simulink model "Drone_2M_sim"  (R2022a)
settings: Solver=VariableStepAuto  StartTime=0.0  StopTime=SIM_TIME  RelTol=1e-3
undefined symbols (not defined in the file or in its folder): batteryMass, batVolt, body, deadCurrent, Dist, footZ, h1al, h1iuse, h1kp, h1td, h1ti, hoverControl, hoverVoltage, hval, hviuse, hvkp, hvtd, hvti, KDrag, Km, Ktrust, minimumMotorVolt, motorMass, paal, pakp, patd, pati, patiuse, pitch_act_lim, propellerMass, pval, pvkp, pvtd, pvti, pvtiuse, Ra, raal, rakp, ral, ratd, rati, ratiuse, rkp, roll_act_lim, roll_limit, rtd, rti, rtiuse, servoUs2Rad, sigbuilder_block, stepPitch, stepRoll, stepYaw, trust_lim, TubeMasse, TubeX, TubeY, UKp, ULimit, UTau_h ... (+49)
libraries: sm_lib x86, nesl_utility x39, sharedtransform x1
(part 1 of 4)
settings Model: Creator=Emar Manla  LastModifiedBy=User
settings DebuggingCC: UnconnectedInputMsg=warning  UnconnectedOutputMsg=warning  UnconnectedLineMsg=warning
settings RTWCC: DLArmComputeVersion=19.05

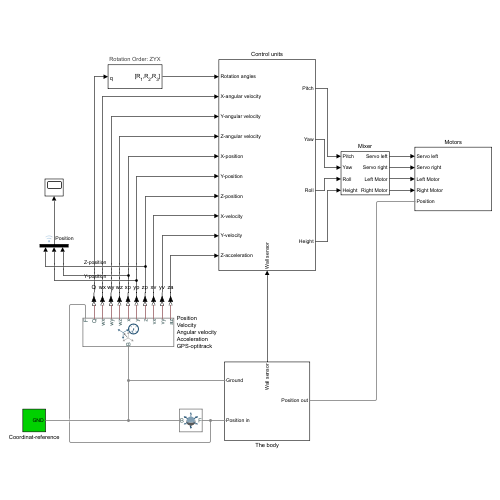
[thumbnail: Simulink's stored preview of the top-level diagram]
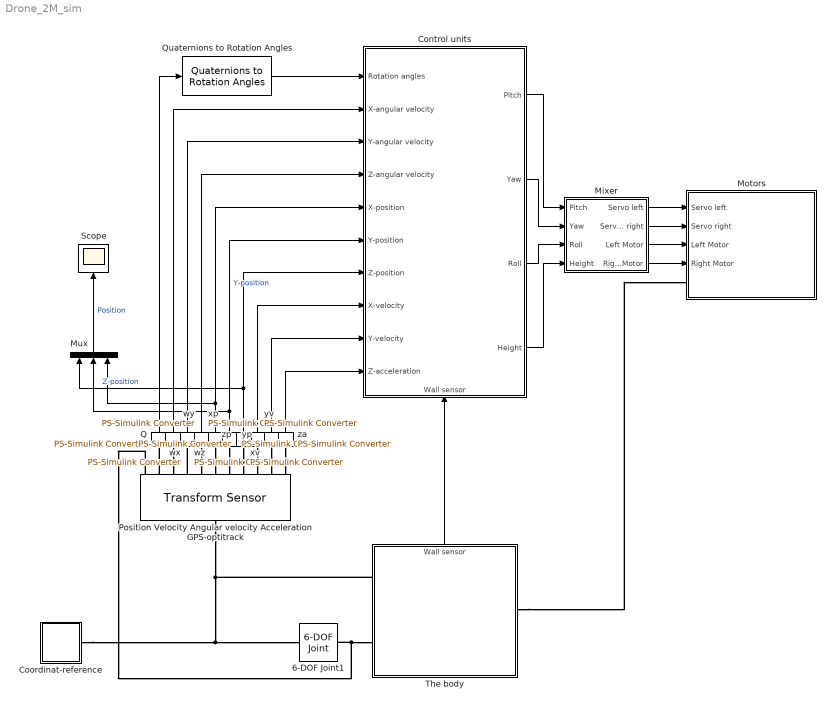
== system Drone_2M_sim ==
  6-DOF Joint1 : sm_lib/Joints/6-DOF Joint  JointMode=Normal  SenseConstraintForce=off  SenseConstraintForceX=off  SenseConstraintForceY=off  SenseConstraintForceZ=off  SenseConstraintTorque=off  SenseConstraintTorqueX=off  SenseConstraintTorqueY=off  SenseConstraintTorqueZ=off  SenseTotalForce=off  SenseTotalForceX=off  SenseTotalForceY=off  SenseTotalForceZ=off  SenseTotalTorque=off  SenseTotalTorqueX=off  SenseTotalTorqueY=off  SenseTotalTorqueZ=off  CompositeWrenchDir=FollowerOnBase  CompositeWrenchFrame=BaseFrame  PxEquilibriumPosition=0  PxEquilibriumPositionUnits=m  PxSpringStiffness=0  PxSpringStiffnessUnits=N/m  PxDampingCoefficient=0  PxDampingCoefficientUnits=N/(m/s)  PxTorqueActuationMode=NoTorque  PxMotionActuationMode=ComputedMotion  PxSensePosition=off  PxSenseVelocity=off  PxSenseAcceleration=off  PxSenseTorqueForce=off  PxSenseLowerLimitTorqueForce=off  PxSenseUpperLimitTorqueForce=off  PxLowerLimitSpecify=off  PxLowerLimitBound=-1  PxLowerLimitBoundUnits=m  PxLowerLimitStiffness=1e6  PxLowerLimitStiffnessUnits=N/m  PxLowerLimitDamping=1e3  PxLowerLimitDampingUnits=N/(m/s)  PxLowerLimitTransitionRegionWidth=1e-4  PxLowerLimitTransitionRegionWidthUnits=m  PxUpperLimitSpecify=off  PxUpperLimitBound=1  PxUpperLimitBoundUnits=m  PxUpperLimitStiffness=1e6  PxUpperLimitStiffnessUnits=N/m  PxUpperLimitDamping=1e3  PxUpperLimitDampingUnits=N/(m/s)  PxUpperLimitTransitionRegionWidth=1e-4  PxUpperLimitTransitionRegionWidthUnits=m  PxPositionTargetSpecify=off  PxPositionTargetPriority=High  PxPositionTargetValue=0  PxPositionTargetValueUnits=m  PxVelocityTargetSpecify=off  PxVelocityTargetPriority=High  PxVelocityTargetValue=0  PxVelocityTargetValueUnits=m/s  PyEquilibriumPosition=0  PyEquilibriumPositionUnits=m  PySpringStiffness=0  PySpringStiffnessUnits=N/m  PyDampingCoefficient=0  PyDampingCoefficientUnits=N/(m/s)  PyTorqueActuationMode=NoTorque  PyMotionActuationMode=ComputedMotion  PySensePosition=off  PySenseVelocity=off  PySenseAcceleration=off  PySenseTorqueForce=off  PySenseLowerLimitTorqueForce=off  PySenseUpperLimitTorqueForce=off  PyLowerLimitSpecify=off  PyLowerLimitBound=-1  PyLowerLimitBoundUnits=m  PyLowerLimitStiffness=1e6  PyLowerLimitStiffnessUnits=N/m  PyLowerLimitDamping=1e3  PyLowerLimitDampingUnits=N/(m/s)  PyLowerLimitTransitionRegionWidth=1e-4  PyLowerLimitTransitionRegionWidthUnits=m  PyUpperLimitSpecify=off  PyUpperLimitBound=1  PyUpperLimitBoundUnits=m  PyUpperLimitStiffness=1e6  PyUpperLimitStiffnessUnits=N/m  PyUpperLimitDamping=1e3  PyUpperLimitDampingUnits=N/(m/s)  PyUpperLimitTransitionRegionWidth=1e-4  PyUpperLimitTransitionRegionWidthUnits=m  PyPositionTargetSpecify=off  PyPositionTargetPriority=High  PyPositionTargetValue=0  PyPositionTargetValueUnits=m  PyVelocityTargetSpecify=off  PyVelocityTargetPriority=High  PyVelocityTargetValue=0  PyVelocityTargetValueUnits=m/s  PzEquilibriumPosition=0  PzEquilibriumPositionUnits=m  PzSpringStiffness=0  PzSpringStiffnessUnits=N/m  PzDampingCoefficient=0  PzDampingCoefficientUnits=N/(m/s)  PzTorqueActuationMode=NoTorque  PzMotionActuationMode=ComputedMotion  PzSensePosition=off  PzSenseVelocity=off  PzSenseAcceleration=off  PzSenseTorqueForce=off  PzSenseLowerLimitTorqueForce=off  PzSenseUpperLimitTorqueForce=off  PzLowerLimitSpecify=off  PzLowerLimitBound=-1  PzLowerLimitBoundUnits=m  PzLowerLimitStiffness=1e6  PzLowerLimitStiffnessUnits=N/m  PzLowerLimitDamping=1e3  PzLowerLimitDampingUnits=N/(m/s)  PzLowerLimitTransitionRegionWidth=1e-4  PzLowerLimitTransitionRegionWidthUnits=m  PzUpperLimitSpecify=off  PzUpperLimitBound=1  PzUpperLimitBoundUnits=m  PzUpperLimitStiffness=1e6  PzUpperLimitStiffnessUnits=N/m  PzUpperLimitDamping=1e3  PzUpperLimitDampingUnits=N/(m/s)  PzUpperLimitTransitionRegionWidth=1e-4  PzUpperLimitTransitionRegionWidthUnits=m  PzPositionTargetSpecify=off  PzPositionTargetPriority=High  PzPositionTargetValue=0  PzPositionTargetValueUnits=m  PzVelocityTargetSpecify=off  PzVelocityTargetPriority=High  PzVelocityTargetValue=0  PzVelocityTargetValueUnits=m/s  SphDefPosRotationMethod=None  SphDefPosRotationAngleUnits=deg  SphDefPosRotationStandardAxis=+Z  SphDefPosRotationAngle=0.0  SphDefPosRotationArbitraryAxis=[0 0 1]  SphDefPosFollAlignAxisA=+X  SphDefPosBaseAlignAxisA=+Y  SphDefPosFollAlignAxisB=+Y  SphDefPosBaseAlignAxisB=+Z  SphDefPosRotationSequenceAxes=FollowerAxes  SphDefPosRotationSequence=XYX  SphDefPosRotationSequenceAngles=[0 0 0]  SphDefPosRotationSequenceAnglesUnits=deg  SphDefPosRotationMatrix=[1 0 0; 0 1 0; 0 0 1]  SphEqPosRotationMethod=None  SphEqPosRotationAngleUnits=deg  SphEqPosRotationStandardAxis=+Z  SphEqPosRotationAngle=0.0  SphEqPosRotationArbitraryAxis=[0 0 1]  SphEqPosFollAlignAxisA=+X  SphEqPosBaseAlignAxisA=+Y  SphEqPosFollAlignAxisB=+Y  SphEqPosBaseAlignAxisB=+Z  SphEqPosRotationSequenceAxes=FollowerAxes  SphEqPosRotationSequence=XYX  SphEqPosRotationSequenceAngles=[0 0 0]  SphEqPosRotationSequenceAnglesUnits=deg  SphEqPosRotationMatrix=[1 0 0; 0 1 0; 0 0 1]  SphSpringStiffness=0  SphSpringStiffnessUnits=N*m/deg  SphDampingCoefficient=0  SphDampingCoefficientUnits=N*m/(deg/s)  SphActuateTorqueX=off  SphActuateTorqueY=off  SphActuateTorqueZ=off  SphActuateTorque=off  SphTorqueActuationMode=NoTorque  SphMotionActuationMode=ComputedMotion  SphActuationFrame=BaseFrame  SphSensePosition=off  SphSenseVelocityX=off  SphSenseVelocityY=off  SphSenseVelocityZ=off  SphSenseVelocity=off  SphSenseAccelerationX=off  SphSenseAccelerationY=off  SphSenseAccelerationZ=off  SphSenseAcceleration=off  SphSenseTorqueX=off  SphSenseTorqueY=off  SphSenseTorqueZ=off  SphSenseTorqueForce=off  SphSenseLowerLimitTorqueMag=off  SphSenseUpperLimitTorqueMag=off  SphSensingFrame=BaseFrame  SphLowerLimitSpecify=off  SphLowerLimitBound=15  SphLowerLimitBoundUnits=deg  SphLowerLimitStiffness=1e4  SphLowerLimitStiffnessUnits=N*m/deg  SphLowerLimitDamping=10  SphLowerLimitDampingUnits=N*m/(deg/s)  SphLowerLimitTransitionRegionWidth=0.1  SphLowerLimitTransitionRegionWidthUnits=deg  SphUpperLimitSpecify=off  SphUpperLimitBound=45  SphUpperLimitBoundUnits=deg  SphUpperLimitStiffness=1e4  SphUpperLimitStiffnessUnits=N*m/deg  SphUpperLimitDamping=10  SphUpperLimitDampingUnits=N*m/(deg/s)  SphUpperLimitTransitionRegionWidth=0.1  SphUpperLimitTransitionRegionWidthUnits=deg  SphPositionTargetRotationMethod=None  SphPositionTargetRotationAngleUnits=deg  SphPositionTargetRotationStandardAxis=+Z  SphPositionTargetRotationAngle=0.0  SphPositionTargetRotationArbitraryAxis=[0 0 1]  SphPositionTargetFollAlignAxisA=+X  SphPositionTargetBaseAlignAxisA=+Y  SphPositionTargetFollAlignAxisB=+Y  SphPositionTargetBaseAlignAxisB=+Z  SphPositionTargetRotationSequenceAxes=FollowerAxes  SphPositionTargetRotationSequence=XYX  SphPositionTargetRotationSequenceAngles=[0 0 0]  SphPositionTargetRotationSequenceAnglesUnits=deg  SphPositionTargetRotationMatrix=[1 0 0; 0 1 0; 0 0 1]  SphPositionTargetSpecify=off  SphPositionTargetPriority=High  SphVelocityTargetValue=[0 0 0]  SphVelocityTargetValueUnits=deg/s  SphVelocityTargetSpecify=off  SphVelocityTargetPriority=High  SphVelocityTargetInFollowerFrame=on
  Control units : Subsystem
      settings: PortSchema="{\"entries\":[{\"content\":{\"sides\":[{\"content\":{\"connectorIds\":[\"In1\",\"In2\",\"In3\",\"In4\",\"In5\",\"In6\",\"In7\",\"In8\",\"In9\",\"In10\"]},\"type\":\"ConnectorPlacement.EquallySpacedRectSide\",\"uuid\":\"d340103e-df0a-4210-bd7d-281fdd84635a\"},{\"content\":{\"connectorIds\":[\"Out1\",\"Out2\",\"Out3\",\"Out4\"],\"side\":\"RIGHT\"},\"type\":\"ConnectorPlacement.EquallySpacedRectSide\",\"uuid\":\"102c7985-49c9-4d2d-a8bd-e75b65b3747e\"},{\"content\":{\"connectorIds\":[],\"side\":\"TOP\"},\"type\":\"ConnectorPlacement.EquallySpacedRectSide\",\"uuid\":\"91d195dd-fb46-4973-a33d-9a570104b146\"},{\"content\":{\"connectorIds\":[\"In11\"],\"side\":\"BOTTOM\"},\"type\":\"ConnectorPlacement.EquallySpacedRectSide\",\"uuid\":\"6514ae44-da82-47f0-9c16-8828a99121c7\"}]},\"type\":\"ConnectorPlacement.EquallySpacedConnector\",\"uuid\":\"d6f0110d-ada7-4d6d-ac5d-6be58cf7ad12\"}],\"packageUris\":[\"http://schema.mathworks.com/mf0/Connector/R2020b\"],\"version\":\"1.0\"}"
  Coordinat-reference : Subsystem
  Mixer : Subsystem
  Motors : Subsystem
  Mux : Mux  Inputs=3
  Position Velocity Angular velocity Acceleration GPS-optitrack : sm_lib/Frames and Transforms/Transform Sensor  MeasurementFrame=World  SenseAngle=off  SenseAxis=off  SenseAngle1=off  SenseAngle2=off  SenseAngle3=off  SenseQ=on  SenseR=off  SenseOmegaX=on  SenseOmegaY=on  SenseOmegaZ=on  SenseOmega1=off  SenseOmega2=off  SenseOmega3=off  SenseQDot=off  SenseRDot=off  SenseAlphaX=off  SenseAlphaY=off  SenseAlphaZ=off  SenseAlpha1=off  SenseAlpha2=off  SenseAlpha3=off  SenseQDDot=off  SenseRDDot=off  SenseX=on  SenseY=on  SenseZ=on  SenseRad=off  SenseAzim=off  SenseDist=off  SenseInc=off  SenseXDot=on  SenseYDot=on  SenseZDot=off  SenseRadDot=off  SenseAzimDot=off  SenseDistDot=off  SenseIncDot=off  SenseXDDot=off  SenseYDDot=off  SenseZDDot=on  SenseRadDDot=off  SenseAzimDDot=off  SenseDistDDot=off  SenseIncDDot=off
  Q : nesl_utility/PS-Simulink Converter  PhysicalDomain=network_engine_domain  SubClassName=ps_output  LeftPortType=input  RightPortType=output  PseudoPeriodic=off  Frequencies=[]  VectorFormat=1-D array  Unit=inherit  AffineConversion=off
      settings: SourceProductBaseCode=SS,PW,VE
  Quaternions to Rotation Angles : sharedtransform/Quaternions to Rotation Angles  rotationOrder=ZYX  aMode=aMode
      settings: SourceProductBaseCode=AE,PW,DR,MT,VE
  Scope : Scope
  The body : Subsystem
      settings: PortSchema="{\"entries\":[{\"content\":{\"sides\":[{\"content\":{\"connectorIds\":[\"LConn1\",\"LConn2\"]},\"type\":\"ConnectorPlacement.EquallySpacedRectSide\",\"uuid\":\"ab37280a-1c0d-4698-b613-0144e6e2cacd\"},{\"content\":{\"connectorIds\":[\"RConn1\"],\"side\":\"RIGHT\"},\"type\":\"ConnectorPlacement.EquallySpacedRectSide\",\"uuid\":\"d03955d5-50d7-455a-845d-681fe8b68e0b\"},{\"content\":{\"connectorIds\":[\"Out1\"],\"side\":\"TOP\"},\"type\":\"ConnectorPlacement.EquallySpacedRectSide\",\"uuid\":\"5fdb51a7-fdf2-45ed-bb3d-bc4d58960f05\"}]},\"type\":\"ConnectorPlacement.EquallySpacedConnector\",\"uuid\":\"890992e6-4a83-43bc-854b-607ea4381fcf\"}],\"packageUris\":[\"http://schema.mathworks.com/mf0/Connector/R2020b\"],\"version\":\"1.0\"}"
  wx : nesl_utility/PS-Simulink Converter  PhysicalDomain=network_engine_domain  SubClassName=ps_output  LeftPortType=input  RightPortType=output  PseudoPeriodic=off  Frequencies=[]  VectorFormat=1-D array  Unit=inherit  AffineConversion=off
      settings: SourceProductBaseCode=SS,PW,VE
  wy : nesl_utility/PS-Simulink Converter  PhysicalDomain=network_engine_domain  SubClassName=ps_output  LeftPortType=input  RightPortType=output  PseudoPeriodic=off  Frequencies=[]  VectorFormat=1-D array  Unit=inherit  AffineConversion=off
      settings: SourceProductBaseCode=SS,PW,VE
  wz : nesl_utility/PS-Simulink Converter  PhysicalDomain=network_engine_domain  SubClassName=ps_output  LeftPortType=input  RightPortType=output  PseudoPeriodic=off  Frequencies=[]  VectorFormat=1-D array  Unit=inherit  AffineConversion=off
      settings: SourceProductBaseCode=SS,PW,VE
  xp : nesl_utility/PS-Simulink Converter  PhysicalDomain=network_engine_domain  SubClassName=ps_output  LeftPortType=input  RightPortType=output  PseudoPeriodic=off  Frequencies=[]  VectorFormat=1-D array  Unit=inherit  AffineConversion=off
      settings: SourceProductBaseCode=SS,PW,VE
  xv : nesl_utility/PS-Simulink Converter  PhysicalDomain=network_engine_domain  SubClassName=ps_output  LeftPortType=input  RightPortType=output  PseudoPeriodic=off  Frequencies=[]  VectorFormat=1-D array  Unit=inherit  AffineConversion=off
      settings: SourceProductBaseCode=SS,PW,VE
  yp : nesl_utility/PS-Simulink Converter  PhysicalDomain=network_engine_domain  SubClassName=ps_output  LeftPortType=input  RightPortType=output  PseudoPeriodic=off  Frequencies=[]  VectorFormat=1-D array  Unit=inherit  AffineConversion=off
      settings: SourceProductBaseCode=SS,PW,VE
  yv : nesl_utility/PS-Simulink Converter  PhysicalDomain=network_engine_domain  SubClassName=ps_output  LeftPortType=input  RightPortType=output  PseudoPeriodic=off  Frequencies=[]  VectorFormat=1-D array  Unit=inherit  AffineConversion=off
      settings: SourceProductBaseCode=SS,PW,VE
  za : nesl_utility/PS-Simulink Converter  PhysicalDomain=network_engine_domain  SubClassName=ps_output  LeftPortType=input  RightPortType=output  PseudoPeriodic=off  Frequencies=[]  VectorFormat=1-D array  Unit=inherit  AffineConversion=off
      settings: SourceProductBaseCode=SS,PW,VE
  zp : nesl_utility/PS-Simulink Converter  PhysicalDomain=network_engine_domain  SubClassName=ps_output  LeftPortType=input  RightPortType=output  PseudoPeriodic=off  Frequencies=[]  VectorFormat=1-D array  Unit=inherit  AffineConversion=off
      settings: SourceProductBaseCode=SS,PW,VE
  wires:
  Q/1 -> Quaternions to Rotation Angles/1
  Mixer/1(Servo left) -> Motors/1(Servo left)
  Mixer/2(Servo right) -> Motors/2(Servo right)
  Mixer/3(Left Motor) -> Motors/3(Left Motor)
  Mixer/4(Right Motor) -> Motors/4(Right Motor)
  Quaternions to Rotation Angles/1 -> Control units/1(Rotation angles)
  xp/1 -> Mux/3, Control units/5(X-position)
  yp/1 -> Mux/2, Control units/6(Y-position)  "Y-position"
  zp/1 -> Mux/1, Control units/7(Z-position)  "Z-position"
  xv/1 -> Control units/8(X-velocity)
  yv/1 -> Control units/9(Y-velocity)
  za/1 -> Control units/10(Z-acceleration)
  wx/1 -> Control units/2(X-angular velocity)
  wy/1 -> Control units/3(Y-angular velocity)
  wz/1 -> Control units/4(Z-angular velocity)
  The body/1(Wall sensor) -> Control units/11(Wall sensor)
  Control units/1(Pitch) -> Mixer/1(Pitch)
  Control units/2(Yaw) -> Mixer/2(Yaw)
  Control units/3(Roll) -> Mixer/3(Roll)
  Control units/4(Height) -> Mixer/4(Height)
  Mux/1 -> Scope/1  "Position"
  connections:
  wx/LConn1 -- Position Velocity Angular velocity Acceleration GPS-optitrack/RConn3
  Position Velocity Angular velocity Acceleration GPS-optitrack/RConn2 -- Q/LConn1
  wz/LConn1 -- Position Velocity Angular velocity Acceleration GPS-optitrack/RConn5
  Position Velocity Angular velocity Acceleration GPS-optitrack/RConn4 -- wy/LConn1
  xp/LConn1 -- Position Velocity Angular velocity Acceleration GPS-optitrack/RConn6
  yp/LConn1 -- Position Velocity Angular velocity Acceleration GPS-optitrack/RConn7
  xv/LConn1 -- Position Velocity Angular velocity Acceleration GPS-optitrack/RConn9
  yv/LConn1 -- Position Velocity Angular velocity Acceleration GPS-optitrack/RConn10
  Position Velocity Angular velocity Acceleration GPS-optitrack/LConn1 -- The body/LConn1 -- Coordinat-reference/RConn1 -- 6-DOF Joint1/LConn1
  Position Velocity Angular velocity Acceleration GPS-optitrack/RConn1 -- The body/LConn2 -- 6-DOF Joint1/RConn1
  The body/RConn1 -- Motors/LConn1
  zp/LConn1 -- Position Velocity Angular velocity Acceleration GPS-optitrack/RConn8
  za/LConn1 -- Position Velocity Angular velocity Acceleration GPS-optitrack/RConn11

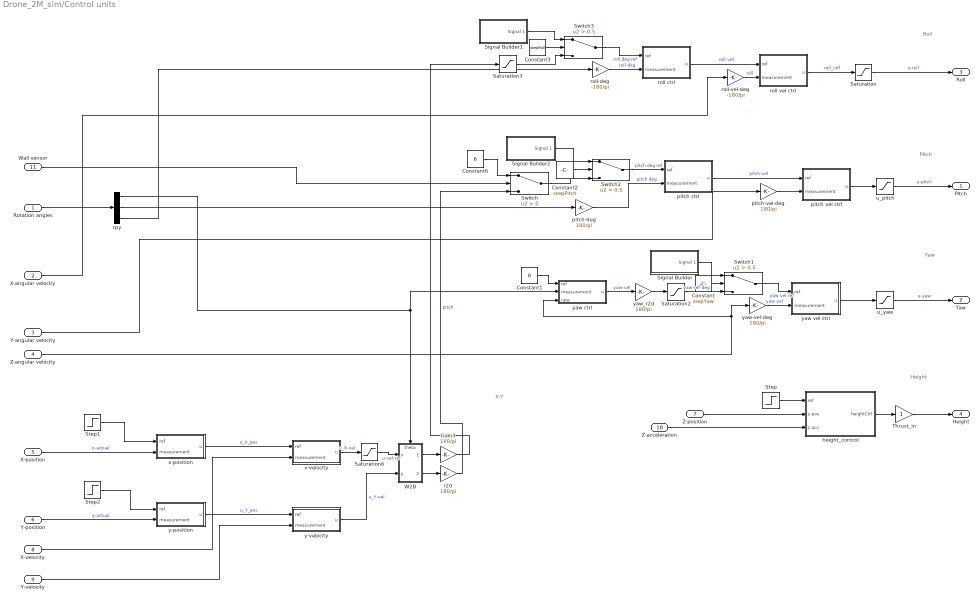
== system Drone_2M_sim/Control units ==
  note: Pitch
  note: Yaw
  note: Roll
  note: Height
  note: X-Y
  Rotation angles : Inport
  X-angular velocity : Inport  Port=2
  Y-angular velocity : Inport  Port=3
  Z-angular velocity : Inport  Port=4
  X-position : Inport  Port=5
  Y-position : Inport  Port=6
  Z-position : Inport  Port=7
  X-velocity : Inport  Port=8
  Y-velocity : Inport  Port=9
  Z-acceleration : Inport  Port=10
  Wall sensor : Inport  Port=11
  Constant : Constant  Value=stepYaw
  Constant1 : Constant  Value=0
  Constant2 : Constant  Value=stepPitch
  Constant3 : Constant  Value=stepRoll
  Constant6 : Constant  Value=6
  Gain3 : Gain  Gain=180/pi
  Saturation : Saturate  UpperLimit=roll_act_lim  LowerLimit=-roll_act_lim
  Saturation2 : Saturate  UpperLimit=yaw_rate_limit  LowerLimit=-yaw_rate_limit
  Saturation3 : Saturate  UpperLimit=roll_limit  LowerLimit=-roll_limit
  Saturation6 : Saturate  UpperLimit=0.008  LowerLimit=-0.008
  Signal Builder : Subsystem  Tag=STV Subsys  LoadFcn=sigbuilder_block('load');  StartFcn=sigbuilder_block('start');  StopFcn=sigbuilder_block('stop');  ClipboardFcn=sigbuilder_block('clipboard');  mask(Sigbuilder block){tuvar=[0:10]}
      mask help: Simulink:masks:SigbuilderBlock_MD
      mask init:
      | if ~strcmp(get_param(bdroot(gcbh),'SimulationStatus'),'stopped') tuvar = sigbuilder_block('maskInit'); end
      settings: CopyFcn=sigbuilder_block('copy');  DeleteFcn=sigbuilder_block('delete');  ModelCloseFcn=sigbuilder_block('modelClose');  PreSaveFcn=sigbuilder_block('preSave');  PauseFcn=sigbuilder_block('pause');  ContinueFcn=sigbuilder_block('continue');  NameChangeFcn=sigbuilder_block('namechange');  OpenFcn=sigbuilder_block('open',[310.5 301 644 239 ]);  CloseFcn=sigbuilder_block('close');
      mask Display: plot(0, 0, 100, 100,[2, 2, 32, 32, 2], [68, 8, 8, 68, 68],[32, 2], [38, 38], [32, 19, 2],[53, 60, 44], [32, 17, 17, 2],[16, 16, 31, 31]);txt = getActiveGroup(gcbh);text(2, 100, txt,'verticalAlignment', 'top');
  Signal Builder1 : Subsystem  Tag=STV Subsys  LoadFcn=sigbuilder_block('load');  StartFcn=sigbuilder_block('start');  StopFcn=sigbuilder_block('stop');  ClipboardFcn=sigbuilder_block('clipboard');  mask(Sigbuilder block){tuvar=[0:10]}
      mask help: Simulink:masks:SigbuilderBlock_MD
      mask init:
      | if ~strcmp(get_param(bdroot(gcbh),'SimulationStatus'),'stopped') tuvar = sigbuilder_block('maskInit'); end
      settings: CopyFcn=sigbuilder_block('copy');  DeleteFcn=sigbuilder_block('delete');  ModelCloseFcn=sigbuilder_block('modelClose');  PreSaveFcn=sigbuilder_block('preSave');  PauseFcn=sigbuilder_block('pause');  ContinueFcn=sigbuilder_block('continue');  NameChangeFcn=sigbuilder_block('namechange');  OpenFcn=sigbuilder_block('open',[310.5 301 644 239 ]);  CloseFcn=sigbuilder_block('close');
      mask Display: plot(0, 0, 100, 100,[2, 2, 32, 32, 2], [68, 8, 8, 68, 68],[32, 2], [38, 38], [32, 19, 2],[53, 60, 44], [32, 17, 17, 2],[16, 16, 31, 31]);txt = getActiveGroup(gcbh);text(2, 100, txt,'verticalAlignment', 'top');
  Signal Builder2 : Subsystem  Tag=STV Subsys  LoadFcn=sigbuilder_block('load');  StartFcn=sigbuilder_block('start');  StopFcn=sigbuilder_block('stop');  ClipboardFcn=sigbuilder_block('clipboard');  mask(Sigbuilder block){tuvar=[0:10]}
      mask help: Simulink:masks:SigbuilderBlock_MD
      mask init:
      | if ~strcmp(get_param(bdroot(gcbh),'SimulationStatus'),'stopped') tuvar = sigbuilder_block('maskInit'); end
      settings: CopyFcn=sigbuilder_block('copy');  DeleteFcn=sigbuilder_block('delete');  ModelCloseFcn=sigbuilder_block('modelClose');  PreSaveFcn=sigbuilder_block('preSave');  PauseFcn=sigbuilder_block('pause');  ContinueFcn=sigbuilder_block('continue');  NameChangeFcn=sigbuilder_block('namechange');  OpenFcn=sigbuilder_block('open',[310.5 301 644 239 ]);  CloseFcn=sigbuilder_block('close');
      mask Display: plot(0, 0, 100, 100,[2, 2, 32, 32, 2], [68, 8, 8, 68, 68],[32, 2], [38, 38], [32, 19, 2],[53, 60, 44], [32, 17, 17, 2],[16, 16, 31, 31]);txt = getActiveGroup(gcbh);text(2, 100, txt,'verticalAlignment', 'top');
  Step : Step  Time=z_steptime  After=z_ref  SampleTime=0
  Step1 : Step  Time=x_steptime  After=x_ref  SampleTime=0
  Step2 : Step  Time=y_steptime  After=y_ref  SampleTime=0
  Switch : Switch  Criteria=u2 > Threshold  SaturateOnIntegerOverflow=off  InputSameDT=off
  Switch1 : Switch  Criteria=u2 > Threshold  Threshold=0.5  SaturateOnIntegerOverflow=off  InputSameDT=off
  Switch2 : Switch  Criteria=u2 > Threshold  Threshold=0.5  SaturateOnIntegerOverflow=off  InputSameDT=off
  Switch3 : Switch  Criteria=u2 > Threshold  Threshold=0.5  SaturateOnIntegerOverflow=off  InputSameDT=off
  Thrust_in : Gain
  W2B : Subsystem
      settings: PortSchema="{\"entries\":[{\"content\":{\"sides\":[{\"content\":{\"connectorIds\":[\"In1\",\"In2\"]},\"type\":\"ConnectorPlacement.EquallySpacedRectSide\",\"uuid\":\"cbb8a801-9e3d-4042-a15f-2b3de221b3e9\"},{\"content\":{\"connectorIds\":[\"Out1\",\"Out2\"],\"side\":\"RIGHT\"},\"type\":\"ConnectorPlacement.EquallySpacedRectSide\",\"uuid\":\"345cd2b8-58a5-4721-b50a-def58b68f03f\"},{\"content\":{\"connectorIds\":[\"In3\"],\"side\":\"TOP\"},\"type\":\"ConnectorPlacement.EquallySpacedRectSide\",\"uuid\":\"a136db43-a3b7-4cbd-bccf-57f3512c0ab6\"}]},\"type\":\"ConnectorPlacement.EquallySpacedConnector\",\"uuid\":\"f3e3d7e3-47e2-471e-9ab4-460d41ed2370\"}],\"packageUris\":[\"http://schema.mathworks.com/mf0/Connector/R2020b\"],\"version\":\"1.0\"}"
  height_control : Subsystem
  pitch ctrl : Subsystem
  pitch vel ctrl : Subsystem
  pitch-deg : Gain  Gain=180/pi
  pitch-vel-deg : Gain  Gain=180/pi
  r2d : Gain  Gain=180/pi
  roll ctrl : Subsystem
  roll vel ctrl : Subsystem
  roll-deg : Gain  Gain=-180/pi
  roll-vel-deg : Gain  Gain=-180/pi
  rpy : Demux  Outputs=3
  u_pitch : Saturate  UpperLimit=pitch_act_lim  LowerLimit=-pitch_act_lim
  u_yaw : Saturate  UpperLimit=yaw_act_lim  LowerLimit=-yaw_act_lim
  x-position : Subsystem
  x-velocity : Subsystem
  y-position : Subsystem
  y-velocity : Subsystem
  yaw ctrl : Subsystem
  yaw vel ctrl : Subsystem
  yaw-vel-deg : Gain  Gain=180/pi
  yaw_r2d : Gain  Gain=180/pi
  Pitch : Outport
  Yaw : Outport  Port=2
  Roll : Outport  Port=3
  Height : Outport  Port=4
  wires:
  Wall sensor/1 -> Switch/2
  pitch-vel-deg/1 -> pitch vel ctrl/2(measurement)
  Step/1 -> height_control/1(ref)
  pitch ctrl/1(u) -> pitch vel ctrl/1(ref)  "pitch-vel"
  rpy/3 -> roll-deg/1
  x-velocity/1(u) -> Saturation6/1  "u_X-vel"
  roll-deg/1 -> roll ctrl/2(measurement)  "roll deg"
  y-position/1(u) -> y-velocity/1(ref)  "u_Y_pos"
  yaw vel ctrl/1(u) -> u_yaw/1
  Saturation6/1 -> W2B/1(x)  "u-vel-ref"
  u_yaw/1 -> Yaw/1  "u-yaw"
  Gain3/1 -> Saturation3/1
  r2d/1 -> Switch/3  "pitch"
  Y-position/1 -> y-position/2(measurement)  "y-actual"
  roll ctrl/1(u) -> roll vel ctrl/1(ref)  "roll-vel"
  u_pitch/1 -> Pitch/1  "u-pitch"
  Saturation/1 -> Roll/1  "u-roll"
  roll-vel-deg/1 -> roll vel ctrl/2(measurement)  "roll"
  x-position/1(u) -> x-velocity/1(ref)  "u_X_pos"
  pitch-deg/1 -> pitch ctrl/2(measurement)  "pitch deg"
  height_control/1(heightCtrl) -> Thrust_in/1
  Constant6/1 -> Switch/1
  roll vel ctrl/1(u) -> Saturation/1  "roll_ctrl"
  Y-velocity/1 -> y-velocity/2(measurement)
  Step2/1 -> y-position/1(ref)
  yaw-vel-deg/1 -> yaw vel ctrl/2(measurement)  "yaw vel"
  rpy/1 -> W2B/3(theta), yaw ctrl/2(measurement)
  yaw ctrl/1(u) -> yaw_r2d/1  "yaw-vel"
  Z-position/1 -> height_control/2(z-pos)
  rpy/2 -> pitch-deg/1
  Y-angular velocity/1 -> pitch-vel-deg/1
  Z-angular velocity/1 -> yaw ctrl/3(rate), yaw-vel-deg/1
  W2B/1(roll) -> Gain3/1
  X-angular velocity/1 -> roll-vel-deg/1
  y-velocity/1(u) -> W2B/2(y)  "u_Y-vel"
  W2B/2(pitch) -> r2d/1
  X-velocity/1 -> x-velocity/2(measurement)
  Z-acceleration/1 -> height_control/3(z-acc)
  pitch vel ctrl/1(u) -> u_pitch/1
  X-position/1 -> x-position/2(measurement)  "x-actual"
  Step1/1 -> x-position/1(ref)
  yaw_r2d/1 -> Saturation2/1
  Rotation angles/1 -> rpy/1
  Thrust_in/1 -> Height/1
  Constant1/1 -> yaw ctrl/1(ref)
  Switch1/1 -> yaw vel ctrl/1(ref)  "yaw vel ref"
  Saturation2/1 -> Switch1/3  "yaw-ref-deg"
  Signal Builder/1(Signal 1) -> Switch1/1
  Saturation3/1 -> Switch3/3
  Signal Builder1/1(Signal 1) -> Switch3/1
  Switch/1 -> Switch2/3
  Switch2/1 -> pitch ctrl/1(ref)  "pitch deg ref"
  Signal Builder2/1(Signal 1) -> Switch2/1
  Constant/1 -> Switch1/2
  Constant2/1 -> Switch2/2
  Constant3/1 -> Switch3/2
  Switch3/1 -> roll ctrl/1(ref)  "roll deg ref"

== system Drone_2M_sim/Coordinat-reference ==
  GroundT : sm_lib/Frames and Transforms/Rigid Transform  TranslationMethod=Cartesian  TranslationStandardOffset=0  TranslationLengthUnit=m  TranslationStandardAxis=+Z  TranslationCartesianOffset=[0 0 0]  TranslationROffset=0  TranslationROffsetUnits=m  TranslationZOffset=0  TranslationZOffsetUnits=m  TranslationThetaOffset=0  TranslationThetaOffsetUnits=deg  RotationMethod=None  RotationAngleUnits=deg  RotationStandardAxis=+Z  RotationAngle=0.0  RotationArbitraryAxis=[0 0 1]  FollAlignAxisA=+X  BaseAlignAxisA=+Y  FollAlignAxisB=+Y  BaseAlignAxisB=+Z  RotationSequenceAxes=FollowerAxes  RotationSequence=XYX  RotationSequenceAngles=[0 0 0]  RotationSequenceAnglesUnits=deg  RotationMatrix=[1 0 0; 0 1 0; 0 0 1]
  Mechanism Configuration : sm_lib/Utilities/Mechanism Configuration  UniformGravity=Constant  GravityVector=[0 0 -9.82]  GravityUnits=m/s^2  LinearizationDelta=0.001  JointModeTransitionNonlinearIterations=2
  Solver Configuration : nesl_utility/Solver Configuration  PhysicalDomain=network_engine_domain  SubClassName=solver  LeftPortType=input  RightPortType=generic  Tones=[]  Harmonics=[]  SimulateNoise=off  Profile=off  UseLocalSampling=off  EnableSwitchedLinearOptims=on  FrequencyDomain=off  UseCCode=off  RelTol=0.001  AbsTol=1e-06  MinStep=1e-09  ToWorkspace=off  RevertToSquareIcSolve=off  NumHomotopyIterations=100  PhasorMode=off  PhasorModeNumHarmonics=1  IndexReductionMethod=DerivativeReplacement  DoDC=off  ResidualTolerance=1e-09  UseLocalSolver=off  LocalSolverChoice=NE_BACKWARD_EULER_ADVANCER  LocalSolverSampleTime=0.001  DoFixedCost=off  MaxNonlinIter=3  MaxModeIter=2  ComputeImpulses=off  ImpulseIterations=2  LinearAlgebra=Sparse  LinearAlgebraNumThread=0  EquationFormulation=NE_TIME_EF  DelaysMemoryBudget=1024  AutomaticFiltering=on  FilteringTimeConstant=0.001  PartitionStorageMethod=AS_NEEDED  PartitionMemoryBudget=1024  PartitionMethod=FAST
      settings: SourceProductBaseCode=SS,PW,VE
  Wall : sm_lib/Body Elements/Brick Solid  GraphicAmbientColor=[0.15 0.15 0.15 1.0]  BasedOnType=Mass  BrickDimensions=[2 0.01 2]  BrickDimensionUnits=m  CenterOfMass=[0 0 0]  CenterOfMassUnits=m  GraphicDiffuseColor=[0.2 0.5 0.2]  Density=1000  DensityUnits=kg/(m^3)  DoExposeReferenceFrame=on  GraphicEmissiveColor=[0.0 0.0 0.0 1.0]  ExportEntireGeometry=off  SerializedFrames=<Frames/>  MarkerShape=Sphere  MarkerSize=10  GraphicType=FromGeometry  InertiaType=CalculateFromGeometry  Mass=1  MassUnits=kg  MomentsOfInertia=[1 1 1]  MomentsOfInertiaUnits=kg*m^2  GraphicOpacity=0.5  ProductsOfInertia=[0 0 0]  ProductsOfInertiaUnits=kg*m^2  GraphicShininess=75  GraphicSpecularColor=[0.5 0.5 0.5 1.0]  GraphicVisPropType=SimpleVisualProperties
  WallT : sm_lib/Frames and Transforms/Rigid Transform  TranslationMethod=Cartesian  TranslationStandardOffset=0  TranslationLengthUnit=m  TranslationStandardAxis=+Z  TranslationCartesianOffset=[1 0 1]  TranslationROffset=0  TranslationROffsetUnits=m  TranslationZOffset=0  TranslationZOffsetUnits=m  TranslationThetaOffset=0  TranslationThetaOffsetUnits=deg  RotationMethod=StandardAxis  RotationAngleUnits=deg  RotationStandardAxis=+Z  RotationAngle=90  RotationArbitraryAxis=[0 0 1]  FollAlignAxisA=+X  BaseAlignAxisA=+Y  FollAlignAxisB=+Y  BaseAlignAxisB=+Z  RotationSequenceAxes=FollowerAxes  RotationSequence=XYX  RotationSequenceAngles=[0 0 0]  RotationSequenceAnglesUnits=deg  RotationMatrix=[1 0 0; 0 1 0; 0 0 1]
  World Frame : sm_lib/Frames and Transforms/World Frame
  ground : sm_lib/Body Elements/Brick Solid  GraphicAmbientColor=[0.15 0.15 0.15 1.0]  BasedOnType=Mass  BrickDimensions=[2 2 0.01]  BrickDimensionUnits=m  CenterOfMass=[0 0 0]  CenterOfMassUnits=m  GraphicDiffuseColor=[0.2 0.5 0.2]  Density=1000  DensityUnits=kg/(m^3)  DoExposeReferenceFrame=on  GraphicEmissiveColor=[0.0 0.0 0.0 1.0]  ExportEntireGeometry=off  SerializedFrames=<Frames/>  MarkerShape=Sphere  MarkerSize=10  GraphicType=FromGeometry  InertiaType=CalculateFromGeometry  Mass=1  MassUnits=kg  MomentsOfInertia=[1 1 1]  MomentsOfInertiaUnits=kg*m^2  GraphicOpacity=1.0  ProductsOfInertia=[0 0 0]  ProductsOfInertiaUnits=kg*m^2  GraphicShininess=75  GraphicSpecularColor=[0.5 0.5 0.5 1.0]  GraphicVisPropType=SimpleVisualProperties
  GND : PMIOPort  Side=Right
  connections:
  Solver Configuration/RConn1 -- GroundT/RConn1 -- GND/RConn1 -- WallT/LConn1 -- World Frame/RConn1 -- Mechanism Configuration/RConn1
  Wall/RConn1 -- WallT/RConn1
  ground/RConn1 -- GroundT/LConn1

== system Drone_2M_sim/Mixer ==
  Pitch : Inport
  Yaw : Inport  Port=2
  Roll : Inport  Port=3
  Height : Inport  Port=4
  Sum19 : Sum  Inputs=+-|
  Sum3 : Sum  Inputs=-+|
  Sum4 : Sum  Inputs=++|
  Sum5 : Sum  Inputs=--|
  Servo left : Outport
  Servo right : Outport  Port=2
  Left Motor : Outport  Port=3
  Right Motor : Outport  Port=4
  wires:
  Yaw/1 -> Sum19/2, Sum5/2
  Height/1 -> Sum4/2, Sum3/2
  Roll/1 -> Sum4/1, Sum3/1
  Sum3/1 -> Left Motor/1
  Pitch/1 -> Sum19/1, Sum5/1
  Sum19/1 -> Servo left/1
  Sum4/1 -> Right Motor/1
  Sum5/1 -> Servo right/1

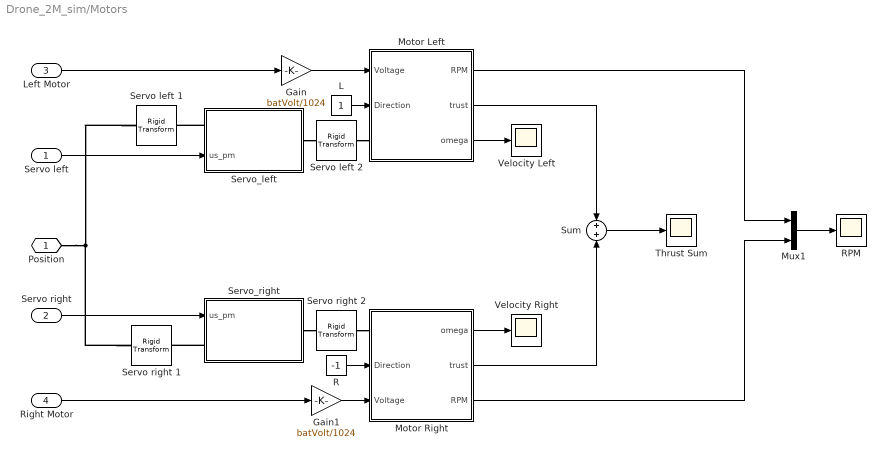
== system Drone_2M_sim/Motors ==
  Servo left : Inport
  Servo right : Inport  Port=2
  Left Motor : Inport  Port=3
  Right Motor : Inport  Port=4
  Gain : Gain  Gain=batVolt/1024
  Gain1 : Gain  Gain=batVolt/1024
  L : Constant
  Motor Left : Subsystem
  Motor Right : Subsystem
      settings: PortSchema="{\"entries\":[{\"content\":{\"sides\":[{\"content\":{\"connectorIds\":[\"LConn1\",\"In1\",\"In2\"]},\"type\":\"ConnectorPlacement.EquallySpacedRectSide\",\"uuid\":\"3ac8ce8c-d7d2-48d4-9826-b935cda4ffeb\"},{\"content\":{\"connectorIds\":[\"Out1\",\"Out2\",\"Out3\"],\"side\":\"RIGHT\"},\"type\":\"ConnectorPlacement.EquallySpacedRectSide\",\"uuid\":\"2c0b9591-3676-4bc5-96fd-efefd902d1a6\"},{\"content\":{\"connectorIds\":[],\"side\":\"TOP\"},\"type\":\"ConnectorPlacement.EquallySpacedRectSide\",\"uuid\":\"2c0b32df-b2c7-4512-ac84-a2a02a011421\"}]},\"type\":\"ConnectorPlacement.EquallySpacedConnector\",\"uuid\":\"47c9c761-0679-463e-a18c-6d64bb0abad1\"}],\"packageUris\":[\"http://schema.mathworks.com/mf0/Connector/R2020b\"],\"version\":\"1.0\"}"
  Mux1 : Mux  Inputs=2
  R : Constant  Value=-1
  RPM : Scope
  Servo left 1 : sm_lib/Frames and Transforms/Rigid Transform  TranslationMethod=StandardAxis  TranslationStandardOffset=-0.2  TranslationLengthUnit=m  TranslationStandardAxis=+Z  TranslationCartesianOffset=[0 0.2 0.03]  TranslationROffset=1  TranslationROffsetUnits=m  TranslationZOffset=0.03  TranslationZOffsetUnits=m  TranslationThetaOffset=-90  TranslationThetaOffsetUnits=deg  RotationMethod=StandardAxis  RotationAngleUnits=deg  RotationStandardAxis=+X  RotationAngle=-45  RotationArbitraryAxis=[0 0 1]  FollAlignAxisA=+X  BaseAlignAxisA=+Y  FollAlignAxisB=+Y  BaseAlignAxisB=+Z  RotationSequenceAxes=FollowerAxes  RotationSequence=XYX  RotationSequenceAngles=[0 0 0]  RotationSequenceAnglesUnits=deg  RotationMatrix=[1 0 0; 0 1 0; 0 0 1]
  Servo left 2 : sm_lib/Frames and Transforms/Rigid Transform  TranslationMethod=None  TranslationStandardOffset=-0.02  TranslationLengthUnit=m  TranslationStandardAxis=+Z  TranslationCartesianOffset=[0 0.2 0.03]  TranslationROffset=1  TranslationROffsetUnits=m  TranslationZOffset=0.03  TranslationZOffsetUnits=m  TranslationThetaOffset=-90  TranslationThetaOffsetUnits=deg  RotationMethod=StandardAxis  RotationAngleUnits=deg  RotationStandardAxis=+X  RotationAngle=45  RotationArbitraryAxis=[0 0 1]  FollAlignAxisA=+X  BaseAlignAxisA=+Y  FollAlignAxisB=+Y  BaseAlignAxisB=+Z  RotationSequenceAxes=FollowerAxes  RotationSequence=XYX  RotationSequenceAngles=[0 0 0]  RotationSequenceAnglesUnits=deg  RotationMatrix=[1 0 0; 0 1 0; 0 0 1]
  Servo right 1 : sm_lib/Frames and Transforms/Rigid Transform  TranslationMethod=StandardAxis  TranslationStandardOffset=-0.2  TranslationLengthUnit=m  TranslationStandardAxis=+Z  TranslationCartesianOffset=[0 0.2 0.03]  TranslationROffset=1  TranslationROffsetUnits=m  TranslationZOffset=0.03  TranslationZOffsetUnits=m  TranslationThetaOffset=-90  TranslationThetaOffsetUnits=deg  RotationMethod=StandardAxis  RotationAngleUnits=deg  RotationStandardAxis=+X  RotationAngle=45  RotationArbitraryAxis=[0 0 1]  FollAlignAxisA=+X  BaseAlignAxisA=+Y  FollAlignAxisB=+Y  BaseAlignAxisB=+Z  RotationSequenceAxes=FollowerAxes  RotationSequence=XYX  RotationSequenceAngles=[0 0 0]  RotationSequenceAnglesUnits=deg  RotationMatrix=[1 0 0; 0 1 0; 0 0 1]
  Servo right 2 : sm_lib/Frames and Transforms/Rigid Transform  TranslationMethod=None  TranslationStandardOffset=-0.02  TranslationLengthUnit=m  TranslationStandardAxis=+Z  TranslationCartesianOffset=[0 0.2 0.03]  TranslationROffset=1  TranslationROffsetUnits=m  TranslationZOffset=0.03  TranslationZOffsetUnits=m  TranslationThetaOffset=-90  TranslationThetaOffsetUnits=deg  RotationMethod=StandardAxis  RotationAngleUnits=deg  RotationStandardAxis=+X  RotationAngle=-45  RotationArbitraryAxis=[0 0 1]  FollAlignAxisA=+X  BaseAlignAxisA=+Y  FollAlignAxisB=+Y  BaseAlignAxisB=+Z  RotationSequenceAxes=FollowerAxes  RotationSequence=XYX  RotationSequenceAngles=[0 0 0]  RotationSequenceAnglesUnits=deg  RotationMatrix=[1 0 0; 0 1 0; 0 0 1]
  Servo_left : Subsystem
      settings: PortSchema="{\"entries\":[{\"content\":{\"sides\":[{\"content\":{\"connectorIds\":[\"LConn1\",\"In1\"]},\"type\":\"ConnectorPlacement.EquallySpacedRectSide\",\"uuid\":\"7755c643-d4e3-4ea5-9f31-089e56e6d032\"},{\"content\":{\"connectorIds\":[\"RConn1\"],\"side\":\"RIGHT\"},\"type\":\"ConnectorPlacement.EquallySpacedRectSide\",\"uuid\":\"44d2886b-f08d-4e92-9ada-ca6df0fa6d88\"},{\"content\":{\"connectorIds\":[],\"side\":\"TOP\"},\"type\":\"ConnectorPlacement.EquallySpacedRectSide\",\"uuid\":\"d2863911-16dd-4ed0-ae3e-c45fa40d1de3\"}]},\"type\":\"ConnectorPlacement.EquallySpacedConnector\",\"uuid\":\"72f1a261-f847-4799-91d8-7adb452c2cfe\"}],\"packageUris\":[\"http://schema.mathworks.com/mf0/Connector/R2020b\"],\"version\":\"1.0\"}"
  Servo_right : Subsystem
  Sum : Sum  Inputs=+|+
  Thrust Sum : Scope
  Velocity Left : Scope
  Velocity Right : Scope
  Position : PMIOPort  Side=Left
  wires:
  Motor Left/3(omega) -> Velocity Left/1
  Motor Left/1(RPM) -> Mux1/1
  Motor Right/1(omega) -> Velocity Right/1
  Motor Right/2(trust) -> Sum/2
  Motor Left/2(trust) -> Sum/1
  Gain1/1 -> Motor Right/2(Voltage)
  R/1 -> Motor Right/1(Direction)
  L/1 -> Motor Left/2(Direction)
  Motor Right/3(RPM) -> Mux1/2
  Servo left/1 -> Servo_left/1(us_pm)
  Mux1/1 -> RPM/1
  Gain/1 -> Motor Left/1(Voltage)
  Left Motor/1 -> Gain/1
  Sum/1 -> Thrust Sum/1
  Servo right/1 -> Servo_right/1(us_pm)
  Right Motor/1 -> Gain1/1
  connections:
  Servo left 1/LConn1 -- Servo right 1/LConn1 -- Position/RConn1
  Servo_right/RConn1 -- Servo right 2/LConn1
  Servo_right/LConn1 -- Servo right 1/RConn1
  Servo right 2/RConn1 -- Motor Right/LConn1
  Servo_left/LConn1 -- Servo left 1/RConn1
  Servo left 2/RConn1 -- Motor Left/LConn1
  Servo_left/RConn1 -- Servo left 2/LConn1
